simulink model "OPEN_LOOP_repeating_sequence"  (Simulink 7.8)
settings: Solver=ode3  StartTime=0.0  StopTime=t_sim  RelTol=1e-3
values from neighbouring files (symbols this model uses):
  baud = 250000    [init.m]    (also in init_101_io_char_up_oloop.m)
  com = 'COM8'    [init.m]    (also in init_101_io_char_up_oloop.m = 'COM33')
  fTf = 0.2    [init.m]    (also in init_101_io_char_up_oloop.m)
  fTl = 0.2    [init.m]    (also in init_101_io_char_up_oloop.m)
  fTt = 0.2    [init.m]    (also in init_101_io_char_up_oloop.m)
  Ts = 0.1    [init.m]    (also in init_101_io_char_up_oloop.m)
libraries: simulink x3, tos_lib x1
settings Model: Creator=tom  LastModifiedBy=kacicak
settings DataIOCC: LimitDataPoints=off
settings DebuggingCC: FcnCallInpInsideContextMsg=Use local settings  StrictBusMsg=Warning

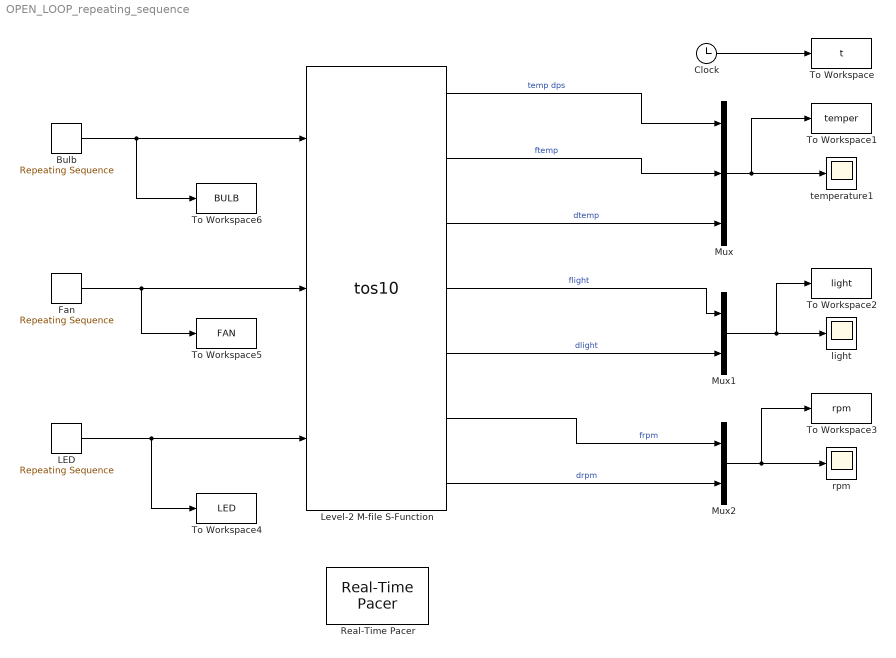
== system OPEN_LOOP_repeating_sequence ==
  Bulb : simulink/Sources/Repeating Sequence  rep_seq_t=TB  rep_seq_y=VB
  Clock : Clock
  Fan : simulink/Sources/Repeating Sequence  rep_seq_t=TF  rep_seq_y=VF
  LED : simulink/Sources/Repeating Sequence  rep_seq_t=TL  rep_seq_y=VL
  Level-2 M-file S-Function : M-S-Function  FunctionName=tos10  Parameters=Ts,com,baud,fTt,fTl,fTf
  Mux : Mux  Inputs=3
  Mux1 : Mux  Inputs=2
  Mux2 : Mux  Inputs=2
  Real-Time Pacer : tos_lib/Real-Time Pacer  simTimePerRealTime=1
  To Workspace : ToWorkspace  VariableName=t  SampleTime=Ts  SaveFormat=Array
  To Workspace1 : ToWorkspace  VariableName=temper  SampleTime=Ts  SaveFormat=Array
  To Workspace2 : ToWorkspace  VariableName=light  SampleTime=Ts  SaveFormat=Array
  To Workspace3 : ToWorkspace  VariableName=rpm  SampleTime=Ts  SaveFormat=Array
  To Workspace4 : ToWorkspace  VariableName=LED  SampleTime=Ts  SaveFormat=Array
  To Workspace5 : ToWorkspace  VariableName=FAN  SampleTime=Ts  SaveFormat=Array
  To Workspace6 : ToWorkspace  VariableName=BULB  SampleTime=Ts  SaveFormat=Array
  light : Scope
      settings: YMax=85  MaxDataPoints=50000
  rpm : Scope
      settings: YMax=85  MaxDataPoints=50000
  temperature1 : Scope
      settings: TimeRange=2400  YMin=-2.5  YMax=45  SaveName=ScopeData4  MaxDataPoints=50000
  wires:
  Bulb/1 -> Level-2 M-file S-Function/1, To Workspace6/1
  Fan/1 -> Level-2 M-file S-Function/2, To Workspace5/1
  LED/1 -> Level-2 M-file S-Function/3, To Workspace4/1
  Mux/1 -> temperature1/1, To Workspace1/1
  Mux1/1 -> light/1, To Workspace2/1
  Clock/1 -> To Workspace/1
  Level-2 M-file S-Function/1 -> Mux/1  "temp dps"
  Level-2 M-file S-Function/2 -> Mux/2  "ftemp"
  Level-2 M-file S-Function/3 -> Mux/3  "dtemp"
  Level-2 M-file S-Function/4 -> Mux1/1  "flight"
  Level-2 M-file S-Function/5 -> Mux1/2  "dlight"
  Level-2 M-file S-Function/7 -> Mux2/2  "drpm"
  Mux2/1 -> To Workspace3/1, rpm/1
  Level-2 M-file S-Function/6 -> Mux2/1  "frpm"
